simulink model "F16_Simulink"  (R2013b)
settings: Solver=ode4  StartTime=0.0  StopTime=10  FixedStep=0.01  RelTol=1e-3
InitFcn:
  | close all; clear; clc;
  | 
  | % Carrega as pastas do sistema
  | MainPath = pwd;
  | Folders = {'Turbina'; 'Atmosfera'; 'Modelo';
  |                  'CoeficientesAerodinamicos'};
  | 
  | for i = 1:numel(Folders)
  |     Pasta = [MainPath '/' Folders{i}];
  |     rmpath(Pasta);
  |     addpath(Pasta);
  | end
  | 
  | % Carrega os valores trimados.
  | load('Trimados.mat');
  | 
  | x0 = x;
values from neighbouring files (symbols this model uses):
  x = [502 0.0370186488564 2.59604154662e-07 0 0.0370186488564 0 0 0 0 0 0 0 ... (13 elements, 1x13)]    [Trimados.mat]
settings Model: Creator=Eduardo  LastModifiedBy=Eduardo

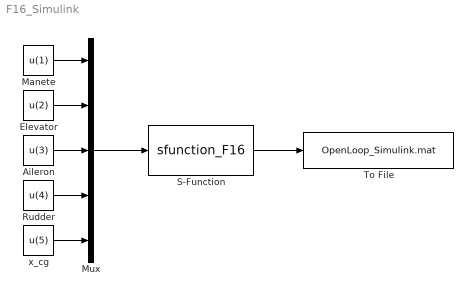
== system F16_Simulink ==
  Aileron : Constant  Value=u(3)
  Elevator : Constant  Value=u(2)
  Manete : Constant  Value=u(1)
  Mux : Mux  Inputs=5
  Rudder : Constant  Value=u(4)
  S-Function : S-Function  FunctionName=sfunction_F16  Parameters=x0  EnableBusSupport=off
  To File : ToFile  Filename=OpenLoop_Simulink.mat  SampleTime=0.01
  x_cg : Constant  Value=u(5)
  wires:
  S-Function/1 -> To File/1
  Rudder/1 -> Mux/4
  Aileron/1 -> Mux/3
  x_cg/1 -> Mux/5
  Manete/1 -> Mux/1
  Mux/1 -> S-Function/1
  Elevator/1 -> Mux/2
